simulink model "Automatisierung_Kapitel8_zustandsregler_Ianteil_beobachter"  (R2015b)
settings: Solver=ode45  StartTime=0.0  StopTime=100  MaxStep=0.2  RelTol=1e-3
values from neighbouring files (symbols this model uses):
  Ac = [0,1,0,0;-1,-1,1,1;0,0,0,1;0.1,0.1,-0.2,-0.2]    [Automatisierung_Kapitel8.m]
  AdL = Ad+kbeo'*cc    [Automatisierung_Kapitel8.m]
  Bc = [bc,bvc]    [Automatisierung_Kapitel8.m]
  BdL = [bd,-kbeo']    [Automatisierung_Kapitel8.m]
  Cc = eye(4)    [Automatisierung_Kapitel8.m]
  CdL = eye(4)    [Automatisierung_Kapitel8.m]
  Dc = [0,0;0,0;0,0;0,0]    [Automatisierung_Kapitel8.m]
  DdL = [0,0;0,0;0,0;0,0]    [Automatisierung_Kapitel8.m]
  kI = ke(5)    [Automatisierung_Kapitel8.m]
  kP = 1/(cc*inv(eye(4)-Ad)*bd)    [Automatisierung_Kapitel8.m]
  kx = kP*cc+ke(1:4)    [Automatisierung_Kapitel8.m]
  Ta = 2    [Automatisierung_Kapitel8.m]
settings Model: Creator=aku  LastModifiedBy=hk
settings DataIOCC: SaveFormat=Array  SignalLoggingSaveFormat=ModelDataLogs
settings OptimizationCC: BooleanDataType=off  ExpressionDepthLimit=2147483647  InitFltsAndDblsToZero=on
settings DebuggingCC: SaveWithParameterizedLinksMsg=none  UnderspecifiedInitializationDetection=Classic  MergeDetectMultiDrivingBlocksExec=none  SignalResolutionControl=TryResolveAllWithWarning  MultiTaskDSMMsg=warning  MultiTaskCondExecSysMsg=none  FcnCallInpInsideContextMsg=EnableAllAsWarning  StateNameClashWarn=warning
settings HardwareCC: ProdBitPerPointer=32  ProdLargestAtomicFloat=None  ProdIntDivRoundTo=Undefined  ProdEndianess=Unspecified  ProdWordSize=32  ProdHWDeviceType=32-bit Generic  TargetUnknown=on
settings GRTTargetCC: TargetFcnLib=ansi_tfl_tmw.mat  GeneratePreprocessorConditionals=Disable all  CombineOutputUpdateFcns=off  GRTInterface=on
settings ConfigComp: CovModelRefEnable=Off  CovSFcnEnable=off

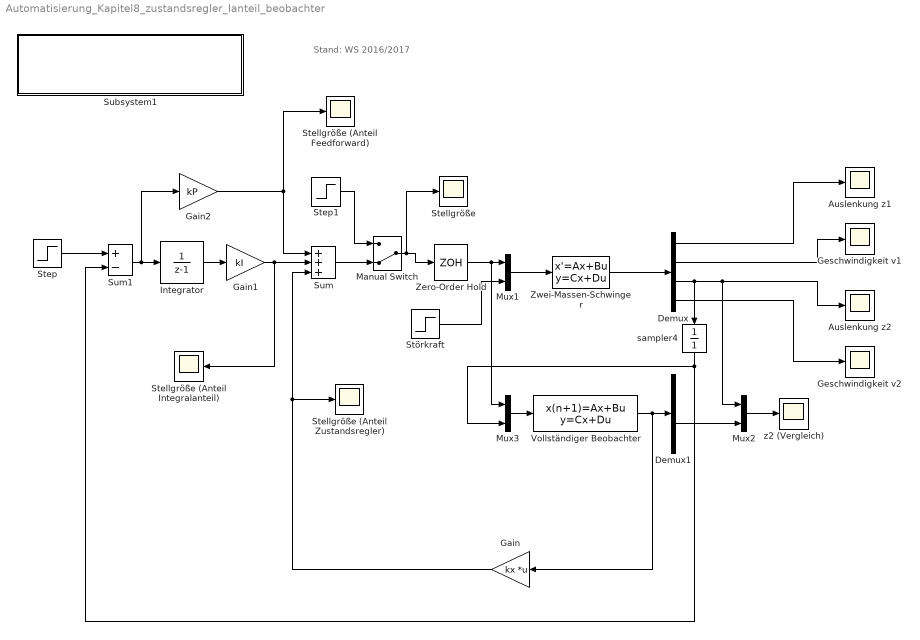
== system Automatisierung_Kapitel8_zustandsregler_Ianteil_beobachter ==
  note: Stand: WS 2016/2017
  Auslenkung z1 : Scope
  Auslenkung z2 : Scope
  Demux : Demux
  Demux1 : Demux
  Gain : Gain  Gain=kx  Multiplication=Matrix(K*u)
  Gain1 : Gain  Gain=kI
  Gain2 : Gain  Gain=kP
  Geschwindigkeit v1 : Scope
  Geschwindigkeit v2 : Scope
  Integrator : DiscreteTransferFcn  Denominator=[1 -1]  SampleTime=Ta
  Manual Switch : ManualSwitch  CurrentSetting=0
  Mux1 : Mux  Inputs=2
  Mux2 : Mux  Inputs=2
  Mux3 : Mux  Inputs=2
  Stellgröße : Scope
  Stellgröße (Anteil Feedforward) : Scope
  Stellgröße (Anteil Integralanteil) : Scope
  Stellgröße (Anteil Zustandsregler) : Scope
  Step : Step  Time=0  SampleTime=0
  Step1 : Step  Time=0  SampleTime=0
  Störkraft : Step  Time=20  SampleTime=0
  Subsystem1 : Subsystem
      settings: OpenFcn=Automatisierung_Kapitel8
      mask Display:
      | disp('Daten laden (Automatisierung_Kapitel8.m)\n\n');
      | disp('(mittels Doppelklick)');
  Sum : Sum  Inputs=+++
  Sum1 : Sum  Inputs=+-
  Vollständiger Beobachter : DiscreteStateSpace  A=AdL  B=BdL  C=CdL  D=DdL  X0=[0,0,0,0]  SampleTime=Ta
  Zero-Order Hold : ZeroOrderHold  SampleTime=Ta
  Zwei-Massen-Schwinger : StateSpace  A=Ac  B=Bc  C=Cc  D=Dc  X0=[0,0,0,0]
  sampler4 : DiscreteTransferFcn  Denominator=[1]  SampleTime=Ta
  z2 (Vergleich) : Scope
  wires:
  Zwei-Massen-Schwinger/1 -> Demux/1
  Mux1/1 -> Zwei-Massen-Schwinger/1
  Zero-Order Hold/1 -> Mux1/1, Mux3/1
  Störkraft/1 -> Mux1/2
  Demux/1 -> Auslenkung z1/1
  Demux/3 -> sampler4/1, Auslenkung z2/1, Mux2/1
  Demux/2 -> Geschwindigkeit v1/1
  Demux/4 -> Geschwindigkeit v2/1
  Gain2/1 -> Sum/1, Stellgröße (Anteil Feedforward)/1
  Sum/1 -> Manual Switch/2
  Manual Switch/1 -> Zero-Order Hold/1, Stellgröße/1
  Step1/1 -> Manual Switch/1
  Step/1 -> Sum1/1
  Sum1/1 -> Integrator/1, Gain2/1
  Gain/1 -> Stellgröße (Anteil Zustandsregler)/1, Sum/3
  Integrator/1 -> Gain1/1
  Gain1/1 -> Sum/2, Stellgröße (Anteil Integralanteil)/1
  Mux3/1 -> Vollständiger Beobachter/1
  Vollständiger Beobachter/1 -> Gain/1, Demux1/1
  sampler4/1 -> Mux3/2, Sum1/2
  Demux1/3 -> Mux2/2
  Mux2/1 -> z2 (Vergleich)/1

== system Automatisierung_Kapitel8_zustandsregler_Ianteil_beobachter/Subsystem1 ==
